simulink model "Lateral_Vehicle_Dynamics_Error_Model"  (R2018a)
settings: Solver=FixedStepAuto  StartTime=0.0  StopTime=1000  FixedStep=0.01  RelTol=1e-3
values from neighbouring files (symbols this model uses):
  C_alpha_f = 80000    [Lateral_Vehicle_Dynamics_Error_Model_Parameters.m]
  C_alpha_r = 80000    [Lateral_Vehicle_Dynamics_Error_Model_Parameters.m]
  Izz = 2873    [Lateral_Vehicle_Dynamics_Error_Model_Parameters.m]
  l_f = 1.58    [Lateral_Vehicle_Dynamics_Error_Model_Parameters.m]
  l_r = 1.58    [Lateral_Vehicle_Dynamics_Error_Model_Parameters.m]
  m = 1000    [Cruise_Control_Simulink_Data.mat]    (also in Lateral_Vehicle_Dynamics_Error_Model_Parameters.m = 1573)
  Vx = 10    [Lateral_Vehicle_Dynamics_Error_Model_Parameters.m]
settings Model: Creator=op95w  LastModifiedBy=op95w

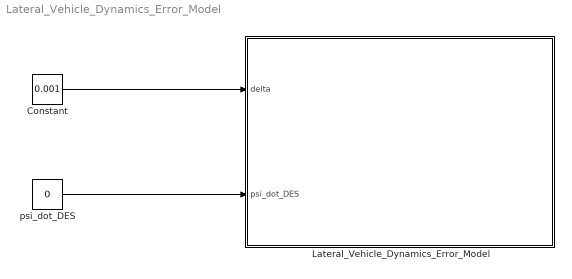
== system Lateral_Vehicle_Dynamics_Error_Model ==
  Constant : Constant  Value=0.001
  Lateral_Vehicle_Dynamics_Error_Model : Subsystem
      mask Display: image(imread('mask1.png'))
  "psi_dot_DES " : Constant  Value=0
  wires:
  "psi_dot_DES "/1 -> Lateral_Vehicle_Dynamics_Error_Model/2(psi_dot_DES)
  Constant/1 -> Lateral_Vehicle_Dynamics_Error_Model/1(delta)

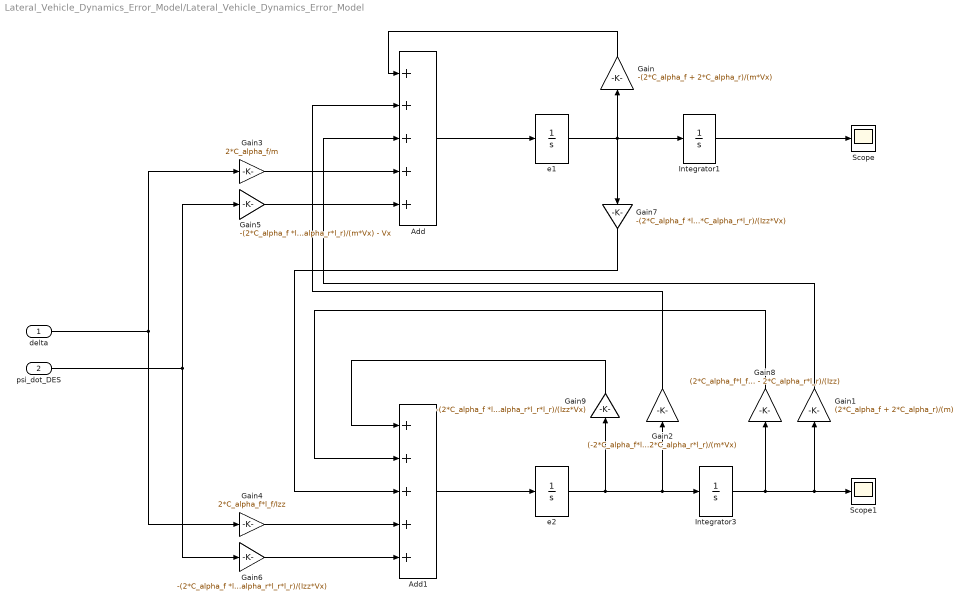
== system Lateral_Vehicle_Dynamics_Error_Model/Lateral_Vehicle_Dynamics_Error_Model ==
  delta : Inport
  psi_dot_DES : Inport  Port=2
  Add : Sum  Inputs=5
  Add1 : Sum  Inputs=5
  Gain : Gain  Gain=-(2*C_alpha_f + 2*C_alpha_r)/(m*Vx)
  Gain1 : Gain  Gain=(2*C_alpha_f + 2*C_alpha_r)/(m)
  Gain2 : Gain  Gain=(-2*C_alpha_f*l_f + 2*C_alpha_r*l_r)/(m*Vx)
  Gain3 : Gain  Gain=2*C_alpha_f/m
  Gain4 : Gain  Gain=2*C_alpha_f*l_f/Izz
  Gain5 : Gain  Gain=-(2*C_alpha_f *l_f - 2*C_alpha_r*l_r)/(m*Vx) - Vx
  Gain6 : Gain  Gain=-(2*C_alpha_f *l_f*l_f+ 2*C_alpha_r*l_r*l_r)/(Izz*Vx)
  Gain7 : Gain  Gain=-(2*C_alpha_f *l_f - 2*C_alpha_r*l_r)/(Izz*Vx)
  Gain8 : Gain  Gain=(2*C_alpha_f*l_f - 2*C_alpha_r*l_r)/(Izz)
  Gain9 : Gain  Gain=-(2*C_alpha_f *l_f*l_f+ 2*C_alpha_r*l_r*l_r)/(Izz*Vx)
  Integrator1 : Integrator
  Integrator3 : Integrator
  Scope : Scope
  Scope1 : Scope
  e1 : Integrator
  e2 : Integrator
  wires:
  e1/1 -> Gain7/1, Gain/1, Integrator1/1
  e2/1 -> Gain9/1, Gain2/1, Integrator3/1
  Gain2/1 -> Add/2
  delta/1 -> Gain3/1, Gain4/1
  psi_dot_DES/1 -> Gain6/1, Gain5/1
  Integrator3/1 -> Gain8/1, Scope1/1, Gain1/1
  Gain6/1 -> Add1/5
  Integrator1/1 -> Scope/1
  Gain9/1 -> Add1/1
  Gain4/1 -> Add1/4
  Gain/1 -> Add/1
  Gain1/1 -> Add/3
  Gain8/1 -> Add1/2
  Gain5/1 -> Add/5
  Add1/1 -> e2/1
  Gain7/1 -> Add1/3
  Add/1 -> e1/1
  Gain3/1 -> Add/4
